simulink model "Torque_Vectoring_Controller"  (R2015a)
settings: Solver=ode4  StartTime=0.0  StopTime=10.0  FixedStep=0.001  RelTol=1e-3
model workspace (MAT data in the model file):
  g = 9.81
  Gr = 10.32
  H = 0.2735
  Krf_a = 183.26
  Krr_a = 325.31
  Ksf = 12153
  Ksr = 14563
  Kwf = 0
  Kwr = 0
  L = 1.525
  Lf = 0.78
  Lr = 0.745
  M = 265
  mu_max = 1.5
  Reff = 0.2325
  Sr = 0.6
  Tf = 1.2
  Tmax = 40
  Tr = 1.2
settings Model: Creator=Michielvdb  LastModifiedBy=Michielvdb

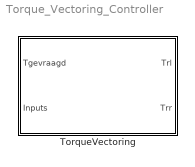
== system Torque_Vectoring_Controller ==
  TorqueVectoring : Subsystem

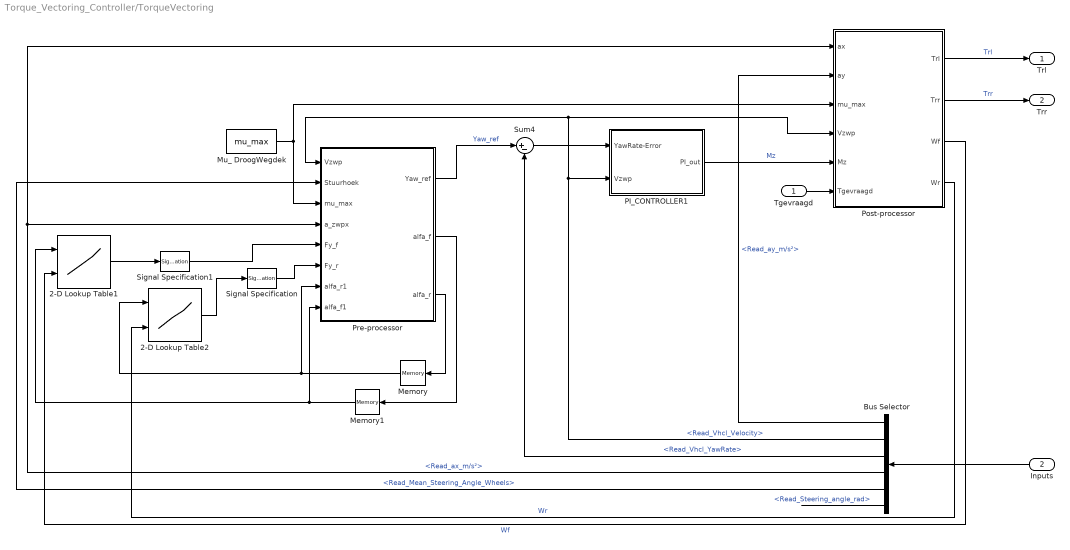
== system Torque_Vectoring_Controller/TorqueVectoring ==
  Tgevraagd : Inport
  Inputs : Inport  Port=2
  2-D Lookup Table1 : Lookup_n-D  BreakpointsForDimension1=[-15,-14,-13,-12,-11,-10,-9,-8,-7,-6,-5,-4,-3,-2,-1,0,1,2,3,4,5,6,7,8,9,10,11,12,13,14,15]  BreakpointsForDimension2=[200,425,650,875,1100]  Table=reshape([-510,-510,-510,-510,-500,-500,-460,-460,-460,-420,-420,-380,-340,-270,-150,0,150,270,340,380,420,420,460,460,460,500,500,500,500,500,500,-1020,-1020,-1020,-1020,-1000,-1000,-1000,-960,-960,-920,-880,-800,-690,-540,-350,0,350,540,690,800,880,920,960,960,1000,1000,1000,1020,1020,1020,1020,-1540,-1540,-1540,-1540,-1500,-1500,-1500,-1460,-1420,-1360,-1300,-1230,-1040,-800,-500,0,500,800,1040,1230,1300,1360,1420,1460,1500,1500,1500,1540,1540,1540,1540,-2020,-2020,-2020,-2020,-1980,-1960,-1920,-1920,-1860,-1790,-1690,-1540,-1330,-960,-580,0,580,960,1330,1540,1690,1790,1860,1920,1920,1960,1980,2020,2020,2020,2020,-2500,-2500,-2500,-2440,-2420,-2420,-2380,-2300,-2250,-2180,-2000,-1800,-1540,-1150,-690,0,690,1150,1540,1800,2000,2180,2250,2300,2380,2420,2420,2440,2500,2500,2500],31,5)  InternalRulePriority=Speed  RndMeth=Simplest  InputSameDT=on
  2-D Lookup Table2 : Lookup_n-D  BreakpointsForDimension1=[-15,-14,-13,-12,-11,-10,-9,-8,-7,-6,-5,-4,-3,-2,-1,0,1,2,3,4,5,6,7,8,9,10,11,12,13,14,15]  BreakpointsForDimension2=[200,425,650,875,1100]  Table=reshape([-510,-510,-510,-510,-500,-500,-460,-460,-460,-420,-420,-380,-340,-270,-150,0,150,270,340,380,420,420,460,460,460,500,500,500,500,500,500,-1020,-1020,-1020,-1020,-1000,-1000,-1000,-960,-960,-920,-880,-800,-690,-540,-350,0,350,540,690,800,880,920,960,960,1000,1000,1000,1020,1020,1020,1020,-1540,-1540,-1540,-1540,-1500,-1500,-1500,-1460,-1420,-1360,-1300,-1230,-1040,-800,-500,0,500,800,1040,1230,1300,1360,1420,1460,1500,1500,1500,1540,1540,1540,1540,-2020,-2020,-2020,-2020,-1980,-1960,-1920,-1920,-1860,-1790,-1690,-1540,-1330,-960,-580,0,580,960,1330,1540,1690,1790,1860,1920,1920,1960,1980,2020,2020,2020,2020,-2500,-2500,-2500,-2440,-2420,-2420,-2380,-2300,-2250,-2180,-2000,-1800,-1540,-1150,-690,0,690,1150,1540,1800,2000,2180,2250,2300,2380,2420,2420,2440,2500,2500,2500],31,5)  InternalRulePriority=Speed  RndMeth=Simplest  InputSameDT=on
  Bus Selector : BusSelector  OutputSignals=Read_ay_m/s²,Read_Vhcl_Velocity,Read_Vhcl_YawRate,Read_ax_m/s²,Read_Mean_Steering_Angle_Wheels,Read_Steering_angle_rad
  Memory : Memory  X0=0.001
  Memory1 : Memory  X0=0.001
  Mu_ DroogWegdek : Constant  Value=mu_max
  PI_CONTROLLER1 : Subsystem
  Post-processor : Subsystem
  Pre-processor : Subsystem
  Signal Specification : SignalSpecification  Dimensions=1
  Signal Specification1 : SignalSpecification  Dimensions=1
  Sum4 : Sum  Inputs=|+-
  Trl : Outport
  Trr : Outport  Port=2
  wires:
  Mu_ DroogWegdek/1 -> Post-processor/3(mu_max), Pre-processor/3(mu_max)
  PI_CONTROLLER1/1(PI_out) -> Post-processor/5(Mz)  "Mz"
  Post-processor/1(Trl) -> Trl/1  "Trl"
  Post-processor/2(Trr) -> Trr/1  "Trr"
  Sum4/1 -> PI_CONTROLLER1/1(YawRate-Error)
  Memory/1 -> Pre-processor/7(alfa_r1), 2-D Lookup Table2/1
  Memory1/1 -> 2-D Lookup Table1/1, Pre-processor/8(alfa_f1)
  Pre-processor/2(alfa_f) -> Memory1/1
  Signal Specification1/1 -> Pre-processor/5(Fy_f)
  Signal Specification/1 -> Pre-processor/6(Fy_r)
  Pre-processor/3(alfa_r) -> Memory/1
  2-D Lookup Table2/1 -> Signal Specification/1
  2-D Lookup Table1/1 -> Signal Specification1/1
  Inputs/1 -> Bus Selector/1
  Tgevraagd/1 -> Post-processor/6(Tgevraagd)
  Bus Selector/6 -> ?  "<Read_Steering_angle_rad>"
  Bus Selector/4 -> Post-processor/1(ax), Pre-processor/4(a_zwpx)  "<Read_ax_m/s²>"
  Bus Selector/1 -> Post-processor/2(ay)  "<Read_ay_m/s²>"
  Bus Selector/2 -> Pre-processor/1(Vzwp), Post-processor/4(Vzwp), PI_CONTROLLER1/2(Vzwp)  "<Read_Vhcl_Velocity>"
  Post-processor/4(Wr) -> 2-D Lookup Table2/2  "Wr"
  Pre-processor/1(Yaw_ref) -> Sum4/1  "Yaw_ref"
  Bus Selector/3 -> Sum4/2  "<Read_Vhcl_YawRate>"
  Post-processor/3(Wf) -> 2-D Lookup Table1/2  "Wf"
  Bus Selector/5 -> Pre-processor/2(Stuurhoek)  "<Read_Mean_Steering_Angle_Wheels>"

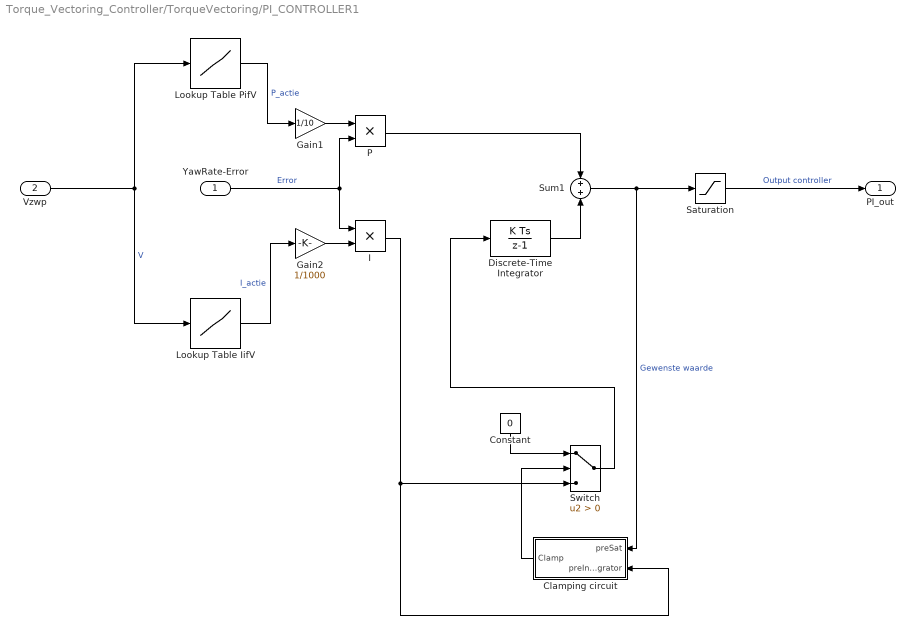
== system Torque_Vectoring_Controller/TorqueVectoring/PI_CONTROLLER1 ==
  YawRate-Error : Inport
  Vzwp : Inport  Port=2
  Clamping circuit : Subsystem
  Constant : Constant  DisableCoverage=on  Value=0  OutDataTypeStr=Inherit: Inherit via back propagation  PreserveConstantTs=on
  Discrete-Time Integrator : DiscreteIntegrator  InitialConditionSetting=State (most efficient)  SampleTime=0.001  LimitOutput=on  UpperSaturationLimit=100  LowerSaturationLimit=-100
  Gain1 : Gain  Gain=1/10
  Gain2 : Gain  Gain=1/1000
  I : Product  RndMeth=Zero
  Lookup Table IifV : Lookup  InputValues=[-1 1 3 5 7 8 10 12 13 15 18 22 26 30 35 40]  Table=[50352886.7892156 50352886.7892156 5589135.45551528 1921428.35851846 975393.735493402 705695.225360316 447460.758905211 279243.629097448 236454.771525978 158654.332416002 94344.5016145154 48661.6461191947 26632.8595225856 13884.3621478696 5589.69756030357 1773.78141835761]
  Lookup Table PifV : Lookup  InputValues=[-1 1 3 5 7 8 10 12 13 15 18 22 26 30 35 40]  Table=[34635.2718980569 34635.2718980569 11590.7926431014 6627.38536761836 4783.12358808128 3932.42492202412 3196.93917901615 2407.06272090184 2253.13792386493 1777.83703218778 1346.39413645714 954.27715290151 744.973517942164 573.513734145603 406.894553185122 261.731683767634]
  P : Product  RndMeth=Zero
  Saturation : Saturate  UpperLimit=500  LowerLimit=-500
  Sum1 : Sum
  Switch : Switch  Criteria=u2 > Threshold  SaturateOnIntegerOverflow=on  InputSameDT=on
  PI_out : Outport
  wires:
  Lookup Table PifV/1 -> Gain1/1  "P_actie"
  Lookup Table IifV/1 -> Gain2/1  "I_actie"
  P/1 -> Sum1/1
  Sum1/1 -> Clamping circuit/1(preSat), Saturation/1  "Gewenste waarde"
  I/1 -> Clamping circuit/2(preIntegrator), Switch/3
  Saturation/1 -> PI_out/1  "Output controller"
  Gain1/1 -> P/1
  YawRate-Error/1 -> P/2, I/1  "Error"
  Vzwp/1 -> Lookup Table PifV/1, Lookup Table IifV/1  "V"
  Gain2/1 -> I/2
  Clamping circuit/1(Clamp) -> Switch/2
  Constant/1 -> Switch/1
  Switch/1 -> Discrete-Time Integrator/1
  Discrete-Time Integrator/1 -> Sum1/2

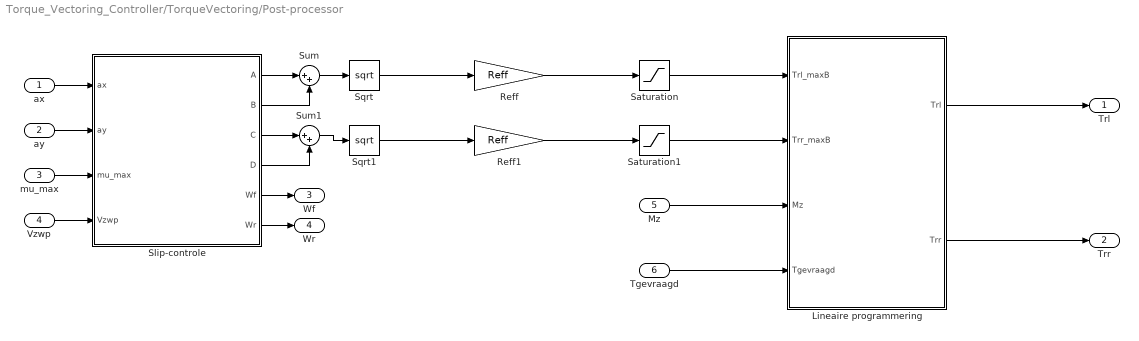
== system Torque_Vectoring_Controller/TorqueVectoring/Post-processor ==
  ax : Inport
  ay : Inport  Port=2
  mu_max : Inport  Port=3
  Vzwp : Inport  Port=4
  Mz : Inport  Port=5
  Tgevraagd : Inport  Port=6
  Lineaire programmering : Subsystem
  Reff : Gain  Gain=Reff
  Reff1 : Gain  Gain=Reff
  Saturation : Saturate  UpperLimit=Gr*Tmax*mu_max  LowerLimit=-Gr*Tmax*mu_max
  Saturation1 : Saturate  UpperLimit=Gr*Tmax*mu_max  LowerLimit=-Gr*Tmax*mu_max
  "Slip-controle " : MATLAB Function  TreatAsAtomicUnit=on
  Sqrt : Sqrt  SaturateOnIntegerOverflow=on
  Sqrt1 : Sqrt  SaturateOnIntegerOverflow=on
  Sum : Sum  Inputs=|++
  Sum1 : Sum  Inputs=|++
  Trl : Outport
  Trr : Outport  Port=2
  Wf : Outport  Port=3
  Wr : Outport  Port=4
  wires:
  Lineaire programmering/2(Trr) -> Trr/1
  Lineaire programmering/1(Trl) -> Trl/1
  Saturation1/1 -> Lineaire programmering/2(Trr_maxB)
  Saturation/1 -> Lineaire programmering/1(Trl_maxB)
  Tgevraagd/1 -> Lineaire programmering/4(Tgevraagd)
  Mz/1 -> Lineaire programmering/3(Mz)
  mu_max/1 -> "Slip-controle "/3(mu_max)
  Vzwp/1 -> "Slip-controle "/4(Vzwp)
  ax/1 -> "Slip-controle "/1(ax)
  ay/1 -> "Slip-controle "/2(ay)
  "Slip-controle "/1(A) -> Sum/1
  "Slip-controle "/3(C) -> Sum1/1
  "Slip-controle "/2(B) -> Sum/2
  "Slip-controle "/4(D) -> Sum1/2
  Sum/1 -> Sqrt/1
  Sum1/1 -> Sqrt1/1
  Sqrt1/1 -> Reff1/1
  Sqrt/1 -> Reff/1
  Reff/1 -> Saturation/1
  Reff1/1 -> Saturation1/1
  "Slip-controle "/6(Wr) -> Wr/1
  "Slip-controle "/5(Wf) -> Wf/1

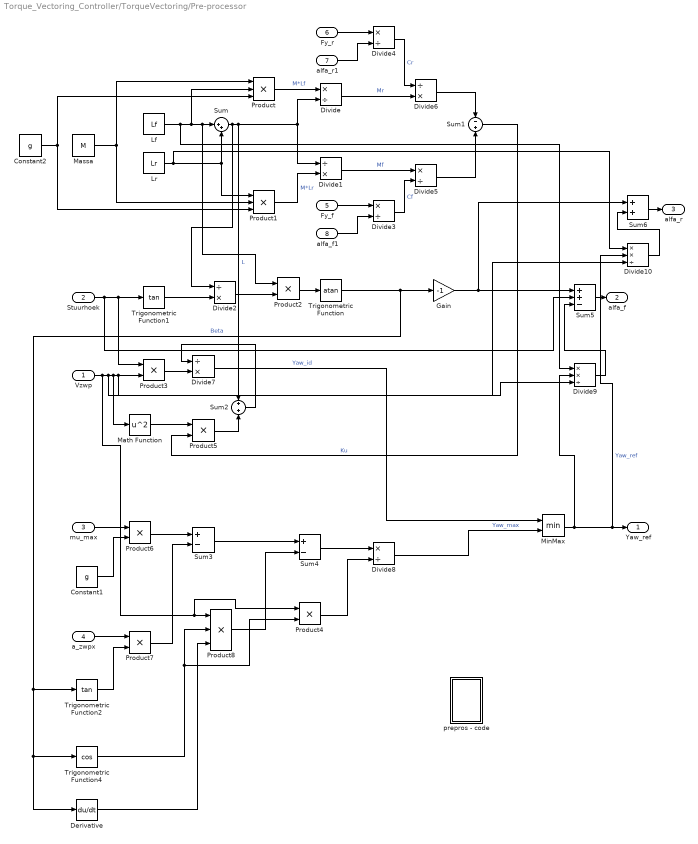
== system Torque_Vectoring_Controller/TorqueVectoring/Pre-processor ==
  Vzwp : Inport
  Stuurhoek : Inport  Port=2
  mu_max : Inport  Port=3
  a_zwpx : Inport  Port=4
  Fy_f : Inport  Port=5
  Fy_r : Inport  Port=6
  alfa_r1 : Inport  Port=7
  alfa_f1 : Inport  Port=8
  Constant1 : Constant  Value=g
  Constant2 : Constant  Value=g
  Derivative : Derivative
  Divide{,3..5,8} (5 alike) : Product  Inputs=*/
  Divide{1..2,6..7} (4 alike) : Product  Inputs=/*
  Divide10 : Product  Inputs=**/
  Divide9 : Product  Inputs=**/
  Gain : Gain  Gain=-1
  Lf : Constant  Value=Lf
  Lr : Constant  Value=Lr
  Massa : Constant  Value=M
  Math Function : Math  Operator=square  SaturateOnIntegerOverflow=on
  MinMax : MinMax  Inputs=2
  Product : Product  Inputs=3
  Product1 : Product  Inputs=3
  Product{2..7} (6 alike) : Product
  Product8 : Product  Inputs=3
  Sum : Sum  Inputs=|++
  Sum1 : Sum  Inputs=-+
  Sum2 : Sum
  Sum3 : Sum  Inputs=+-
  Sum4 : Sum  Inputs=+-
  Sum5 : Sum  Inputs=++-
  Sum6 : Sum
  Trigonometric Function : Trigonometry  Operator=atan
  Trigonometric Function1 : Trigonometry  Operator=tan
  Trigonometric Function2 : Trigonometry  Operator=tan
  Trigonometric Function4 : Trigonometry  Operator=cos
  prepros - code : Subsystem
  Yaw_ref : Outport
  alfa_f : Outport  Port=2
  alfa_r : Outport  Port=3
  wires:
  Product8/1 -> Sum4/2
  Product4/1 -> Divide8/2
  Derivative/1 -> Product8/3
  MinMax/1 -> Divide9/2, Divide10/2, Yaw_ref/1  "Yaw_ref"
  Divide8/1 -> MinMax/2  "Yaw_max"
  Sum4/1 -> Divide8/1
  Fy_r/1 -> Divide4/1
  Divide4/1 -> Divide6/1  "Cr"
  Divide6/1 -> Sum1/1
  Trigonometric Function1/1 -> Divide2/2
  Divide1/1 -> Divide5/1  "Mf"
  Divide2/1 -> Product2/2
  alfa_f1/1 -> Divide3/2
  Divide/1 -> Divide6/2  "Mr"
  Trigonometric Function/1 -> Gain/1, Trigonometric Function2/1, Derivative/1, Trigonometric Function4/1  "Beta"
  alfa_r1/1 -> Divide4/2
  Product1/1 -> Divide1/2  "M*Lr"
  Lf/1 -> Divide9/1, Product/2, Product2/1, Sum/1
  Product2/1 -> Trigonometric Function/1
  Divide3/1 -> Divide5/2  "Cf"
  Massa/1 -> Product/1, Product1/2
  Product/1 -> Divide/1  "M*Lf"
  Sum/1 -> Divide/2, Divide1/1, Sum2/1, Divide2/1  "L"
  Lr/1 -> Divide10/1, Product1/1, Sum/2
  Math Function/1 -> Product5/1
  mu_max/1 -> Product6/1
  Trigonometric Function4/1 -> Product4/2, Product8/2
  Product5/1 -> Sum2/2
  Product6/1 -> Sum3/1
  Constant1/1 -> Product6/2
  Sum1/1 -> Product5/2  "Ku"
  Divide7/1 -> MinMax/1  "Yaw_id"
  Product7/1 -> Sum3/2
  Sum3/1 -> Sum4/1
  Divide5/1 -> Sum1/2
  Sum2/1 -> Divide7/1
  Vzwp/1 -> Product4/1, Product8/1, Divide9/3, Math Function/1, Divide10/3, Product3/2
  Trigonometric Function2/1 -> Product7/2
  a_zwpx/1 -> Product7/1
  Product3/1 -> Divide7/2
  Gain/1 -> Sum6/1, Sum5/1
  Divide9/1 -> Sum5/3
  Sum5/1 -> alfa_f/1
  Divide10/1 -> Sum6/2
  Sum6/1 -> alfa_r/1
  Constant2/1 -> Product1/3, Product/3
  Fy_f/1 -> Divide3/1
  Stuurhoek/1 -> Sum5/2, Product3/1, Trigonometric Function1/1

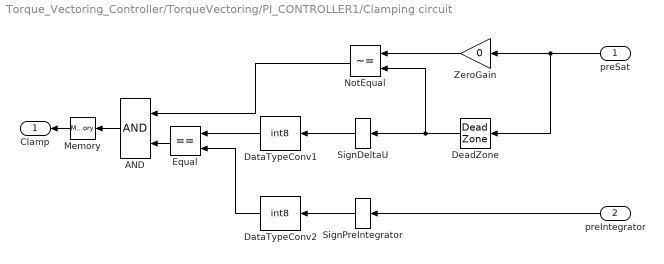
== system Torque_Vectoring_Controller/TorqueVectoring/PI_CONTROLLER1/Clamping circuit ==
  preSat : Inport  DisableCoverage=on
  preIntegrator : Inport  DisableCoverage=on  Port=2
  AND : Logic  DisableCoverage=on
  DataTypeConv1 : DataTypeConversion  DisableCoverage=on  OutDataTypeStr=int8  SaturateOnIntegerOverflow=on  RndMeth=Zero  LockScale=on
  DataTypeConv2 : DataTypeConversion  DisableCoverage=on  OutDataTypeStr=int8  SaturateOnIntegerOverflow=on  RndMeth=Zero  LockScale=on
  DeadZone : DeadZone  DisableCoverage=on  LowerValue=-100  UpperValue=100  SaturateOnIntegerOverflow=on
  Equal : RelationalOperator  DisableCoverage=on  Operator===  InputSameDT=on
  Memory : Memory  DisableCoverage=on
  NotEqual : RelationalOperator  DisableCoverage=on  Operator=~=  InputSameDT=on
  SignDeltaU : Signum  DisableCoverage=on
  SignPreIntegrator : Signum  DisableCoverage=on
  ZeroGain : Gain  DisableCoverage=on  Gain=0  SaturateOnIntegerOverflow=on  OutDataTypeStr=Inherit: Same as input  ParamDataTypeStr=Inherit: Same as input
  Clamp : Outport  DisableCoverage=on
  wires:
  preSat/1 -> ZeroGain/1, DeadZone/1
  preIntegrator/1 -> SignPreIntegrator/1
  ZeroGain/1 -> NotEqual/1
  DeadZone/1 -> NotEqual/2, SignDeltaU/1
  SignDeltaU/1 -> DataTypeConv1/1
  DataTypeConv1/1 -> Equal/1
  SignPreIntegrator/1 -> DataTypeConv2/1
  DataTypeConv2/1 -> Equal/2
  NotEqual/1 -> AND/1
  Equal/1 -> AND/2
  AND/1 -> Memory/1
  Memory/1 -> Clamp/1

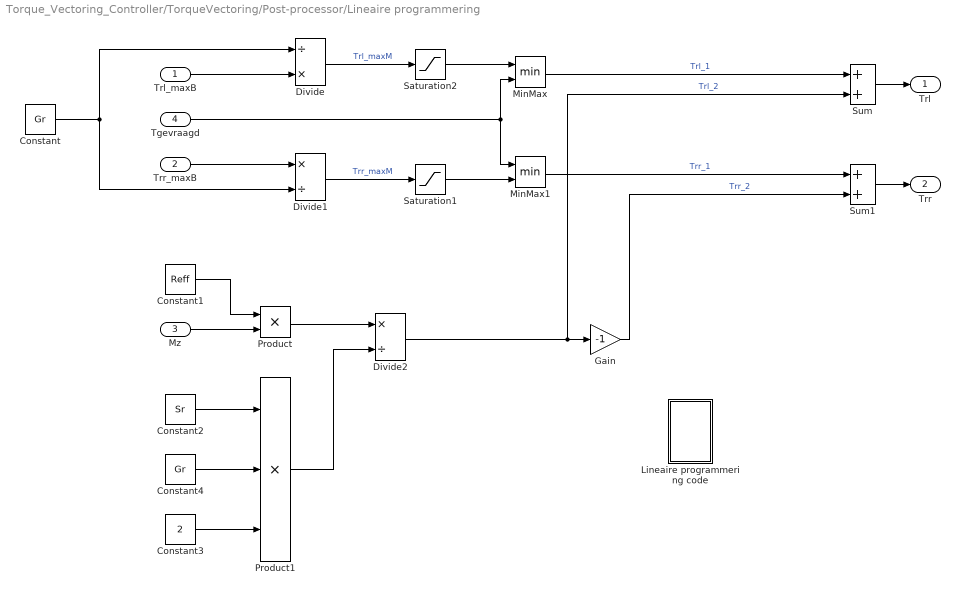
== system Torque_Vectoring_Controller/TorqueVectoring/Post-processor/Lineaire programmering ==
  Trl_maxB : Inport
  Trr_maxB : Inport  Port=2
  Mz : Inport  Port=3
  Tgevraagd : Inport  Port=4
  Constant : Constant  Value=Gr
  Constant1 : Constant  Value=Reff
  Constant2 : Constant  Value=Sr
  Constant3 : Constant  Value=2
  Constant4 : Constant  Value=Gr
  Divide : Product  Inputs=/*
  Divide1 : Product  Inputs=*/
  Divide2 : Product  Inputs=*/
  Gain : Gain  Gain=-1
  Lineaire programmering code : Subsystem
  MinMax : MinMax  Inputs=2
  MinMax1 : MinMax  Inputs=2
  Product : Product
  Product1 : Product  Inputs=3
  Saturation1 : Saturate  UpperLimit=Tmax  LowerLimit=-Tmax
  Saturation2 : Saturate  UpperLimit=Tmax  LowerLimit=-Tmax
  Sum : Sum
  Sum1 : Sum
  Trl : Outport
  Trr : Outport  Port=2
  wires:
  Divide/1 -> Saturation2/1  "Trl_maxM"
  Trr_maxB/1 -> Divide1/1
  Constant2/1 -> Product1/1
  Product/1 -> Divide2/1
  Product1/1 -> Divide2/2
  Divide2/1 -> Gain/1, Sum/2  "Trl_2"
  Constant1/1 -> Product/1
  Sum1/1 -> Trr/1
  Constant4/1 -> Product1/2
  MinMax/1 -> Sum/1  "Trl_1"
  MinMax1/1 -> Sum1/1  "Trr_1"
  Constant/1 -> Divide/1, Divide1/2
  Trl_maxB/1 -> Divide/2
  Tgevraagd/1 -> MinMax1/1, MinMax/2
  Gain/1 -> Sum1/2  "Trr_2"
  Constant3/1 -> Product1/3
  Sum/1 -> Trl/1
  Mz/1 -> Product/2
  Divide1/1 -> Saturation1/1  "Trr_maxM"
  Saturation2/1 -> MinMax/1
  Saturation1/1 -> MinMax1/2

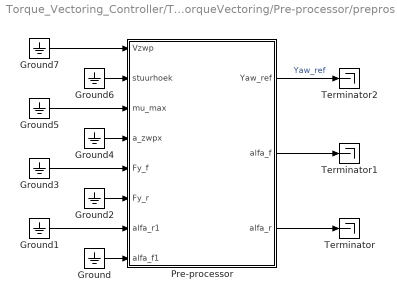
== system Torque_Vectoring_Controller/TorqueVectoring/Pre-processor/prepros - code ==
  Ground{,1..7} (8 alike) : Ground
  Pre-processor : MATLAB Function  TreatAsAtomicUnit=on
  Terminator : Terminator
  Terminator1 : Terminator
  Terminator2 : Terminator
  wires:
  Pre-processor/2(alfa_f) -> Terminator1/1
  Ground2/1 -> Pre-processor/6(Fy_r)
  Ground7/1 -> Pre-processor/1(Vzwp)
  Ground5/1 -> Pre-processor/3(mu_max)
  Ground/1 -> Pre-processor/8(alfa_f1)
  Ground1/1 -> Pre-processor/7(alfa_r1)
  Pre-processor/3(alfa_r) -> Terminator/1
  Pre-processor/1(Yaw_ref) -> Terminator2/1  "Yaw_ref"
  Ground3/1 -> Pre-processor/5(Fy_f)
  Ground6/1 -> Pre-processor/2(stuurhoek)
  Ground4/1 -> Pre-processor/4(a_zwpx)

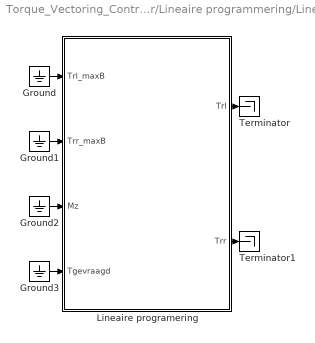
== system Torque_Vectoring_Controller/TorqueVectoring/Post-processor/Lineaire programmering/Lineaire programmering code ==
  Ground{,1..3} (4 alike) : Ground
  Lineaire programering : MATLAB Function  TreatAsAtomicUnit=on
  Terminator : Terminator
  Terminator1 : Terminator
  wires:
  Lineaire programering/2(Trr) -> Terminator1/1
  Lineaire programering/1(Trl) -> Terminator/1
  Ground/1 -> Lineaire programering/1(Trl_maxB)
  Ground2/1 -> Lineaire programering/3(Mz)
  Ground3/1 -> Lineaire programering/4(Tgevraagd)
  Ground1/1 -> Lineaire programering/2(Trr_maxB)

== matlab function Torque_Vectoring_Controller/TorqueVectoring/Post-processor/Lineaire programmering/Lineaire programmering code/Lineaire programering ==
  data: Trl_maxB input; Trl output; Trr_maxB input; Mz input; Tgevraagd input; Trr output
function [Trl,Trr] = Lineaire_programmering(Trl_maxB,Trr_maxB,Mz,Tgevraagd)
%Dit blok staat in voor het berekenen van het te leveren koppel per wiel
%aan de hand van twee lineaire doelen. Het eerste doel is het gewenst 
%koppel om rechtdoor te rijden. Het tweede doel is het berekende moment van 
%de PI-regelaar om te zetten naar een koppelverschil van maximaal 10 Nm 
%over de twee achterwielen.
%Als de twee doelen berekend zijn worden ze opgeteld om tot het
%resulterende koppel per wiel te komen. Deze koppels worden naar het
%wagenmodel of de motordrives van de effectieve wagen gestuurd.

%%
%Parameters
Reff	=0.2325;            
Gr      =10.32;             
Sr      =0.600;                 

%%
%Eerste versie

%Gevraagd koppel rechtdoor
Trl_maxM = Trl_maxB/Gr;
Trr_maxM = Trr_maxB/Gr;

Trl_1 = min(Trl_maxM,Tgevraagd);
Trr_1 = min(Trr_maxM,Tgevraagd);

%Gevraagd moment om z-as
T_delta = (Mz*Reff)/(2*Sr*Gr) ;

Trl_2 = T_delta;
Trr_2 = -T_delta;

%Totaal koppel
Trl = Trl_1 + Trl_2;
Trr = Trr_1 + Trr_2;

== matlab function Torque_Vectoring_Controller/TorqueVectoring/Post-processor/Slip-controle  ==
  data: ax input; ay input; mu_max input; A output; Vzwp input; B output; C output; D output; Wf output; Wr output
function [A,B,C,D,Wf,Wr] = Slip_controle(ax,ay,mu_max,Vzwp)
% Berekening van de maximale torques die men kan toepassen op de wielen
% door berekening van de normaalkrachten op de wielen.

%load('parameters.mat');

M       = 265;             
L       = 1.525;                           
Lf      = 0.780;                              
Lr      = 0.745;                              
Tf      = 1.200;                             
Tr      = 1.200;                            
g       = 9.81;                                                       
Krf_a	= 183.26;                            
Krr_a	= 325.31;                           
Ksf     = 12153;             %Veerstijfheid vooraan
Ksr     = 14563;
H       = 0.2735;                        
    %ax      =0;                 
    %ay      =0;                               
    %Vzwp    =0;                 
    %mu_max  =1.5;

%Wielbelastingen

%Statische wielbelasting
Ws_fl = ((Lr*M*g)/(2*L));
Ws_fr = ((Lr*M*g)/(2*L));
Ws_rl = ((Lf*M*g)/(2*L));
Ws_rr = ((Lf*M*g)/(2*L));

%Ws_f = Ws_fl + Ws_fr;
%Ws_r = Ws_rl + Ws_rr;

%Laterale wielbelasting (door rollen van de wagen)
Wy_fl = -((H*M*ay)/(2*Tf));                         %Kracht per wiel
Wy_fr =  ((H*M*ay)/(2*Tf));
Wy_rl = -((H*M*ay)/(2*Tr));
Wy_rr =  ((H*M*ay)/(2*Tr));

%Longitudinale wielbelasting
Wx_fl = -((H*M*ax)/(2*L));                          %Kracht per wiel
Wx_fr = -((H*M*ax)/(2*L));
Wx_rl =  ((H*M*ax)/(2*L));
Wx_rr =  ((H*M*ax)/(2*L));

%Aerodynamische wielbelasting
LF = -0.0237*(Vzwp)^2 + 0.0958*Vzwp;                %Nog na te kijken; komt uit excel van aeromannen
LR = -0.0237*(Vzwp)^2 + 0.0958*Vzwp;                %Nog na te kijken; komt uit excel van aeromannen

Wa_fl = (-LF/2);  %+((Krf/(Krf+Krr))*(Rm/Tf));      %is er hier 2x rolmoment??? (zie lateraal)
Wa_fr = (-LF/2);  %-((Krf/(Krf+Krr))*(Rm/Tf));
Wa_rl = (-LR/2);  %+((Krr/(Krf+Krr))*(Rm/Tr));
Wa_rr = (-LR/2);  %-((Krr/(Krf+Krr))*(Rm/Tr));

%anti-roll bar wielbelasting
Wab_fl =  ((Krf_a*(-Wy_fl))/((Krf_a+((Ksf*(Tf)^2)/2))));
Wab_fr =  ((Krf_a*(-Wy_fr))/((Krf_a+((Ksf*(Tf)^2)/2))));
Wab_rl =  ((Krr_a*(-Wy_rl))/((Krr_a+((Ksr*(Tr)^2)/2))));
Wab_rr =  ((Krr_a*(-Wy_rr))/((Krr_a+((Ksr*(Tr)^2)/2))));

%Totale belasting per wiel
Wfl = Ws_fl + Wy_fl + Wx_fl + Wa_fl + Wab_fl;   %Ongebruikt, kan later eventueel gebruikt worden voor 4WD??
Wfr = Ws_fr + Wy_fr + Wx_fr + Wa_fr + Wab_fr;   %^ Idem
Wrl = Ws_rl + Wy_rl + Wx_rl + Wa_rl + Wab_rl;
Wrr = Ws_rr + Wy_rr + Wx_rr + Wa_rr + Wab_rr;



%%Omrekening naar torques
%HIER GEWIJZIGD

%Wrijvingscirkels (wortels worden naar buiten gebracht; kunnen niet
%berekend worden in code; geeft fouten; vervolgens ook vermenigvuldigen 
%met effectieve bandenstraal om tot de wielkoppels te komen)

%Jx_rl = ((Wrl*mu_max)^2-((Wrl*ay)/(g))^2);
%Jx_rr = ((Wrr*mu_max)^2-((Wrr*ay)/(g))^2);

%     if Jx_rl < 0
%     then Jx_rl = 0
% end
% 
% if Jx_rr < 0
%     then Jx_rr = 0
% end


A = (Wrl*mu_max)^2;
B = ((Wrl*ay)/(g))^2;
C = (Wrr*mu_max)^2;
D = ((Wrr*ay)/(g))^2;

% Fx_rl = sqrt((Wrl*mu_max)^2-((Wrl*ay)/(g))^2);
% 
% Fx_rr = sqrt((Wrr*mu_max)^2-((Wrr*ay)/(g))^2);

%Maximum torques
% Trl_max = Fx_rl*Reff;
% Trr_max = Fx_rr*Reff;

%Belastingen per as
Wf = (Wfl+Wfr)/2;
Wr = (Wrl+Wrr)/2;

== matlab function Torque_Vectoring_Controller/TorqueVectoring/Pre-processor/prepros - code/Pre-processor ==
  data: Yaw_ref output; Vzwp input; stuurhoek input; mu_max input; a_zwpx input; Fy_f input; Fy_r input; alfa_r1 input; alfa_f output; alfa_r output; alfa_f1 input
function [Yaw_ref,alfa_f,alfa_r]= pre_processor(Vzwp,stuurhoek,mu_max,a_zwpx,Fy_f,Fy_r,alfa_r1,alfa_f1)
%De pre-processor berekend de gewenste yaw rate door het minimum te nemen
%van de ideale en de maximale yaw rate waarde.
%Belangrijk hierbij de hoeken in RAD!!!!!!

%Parameters
M       = 265;             
L       = 1.525;                           
Lf      = 0.780;                              
Lr      = 0.745; 
g       = 9.81;

%Berekening massa's
Wf = (M*Lr*g/L);
Wr = (M*Lf*g/L);

% berekening van de sliphoek beita
beita = atan(Lf * tan(stuurhoek)/ (Lf+Lr)) ;



%Berekening Cornering stiffness
               Cf = (Fy_f/alfa_f1);
               Cr = (Fy_r/alfa_r1);
%              C_rl = (Fy_rl/alfa_rl);
%              C_rr = (Fy_rr/alfa_rr);
                
 % Fy_f = Cf * alfa_f ;
 % Fy_r = Cr * alfa_r ;
%Gemiddelde van de cornering stiffness vooraan en achteraan nemen
          %Cf = ((C_fl + C_fr)/ 2);
          %Cr = ((C_rl + C_rr)/ 2);
%Berekening van de onderstuur factor.
Ku = ((Wf/Cf)-(Wr/Cr));

%Berekening van de ideale yaw rate.
Yaw_id = ((Vzwp*stuurhoek)/((Lf+Lr)+Ku*(Vzwp)^2));

%Berekening van de maximale yaw rate.
Yaw_max = (((mu_max*g)-(a_zwpx * tan(beita)) - (Vzwp * cos(beita)* diff(beita)))/(Vzwp*cos(beita)));

%Minimale yaw rate.
Yaw_ref = min([Yaw_id ; Yaw_max]);
%Berekening sliphoeken
alfa_f = - beita + stuurhoek - ((Lf * Yaw_ref)/Vzwp);
alfa_r = - beita + ((Lr * Yaw_ref)/Vzwp);
